simulink model "qiita2"  (R2019a)
settings: Solver=FixedStepDiscrete  StartTime=0.0  StopTime=Inf  FixedStep=0.001  RelTol=1e-3  EnableMultiTasking=on
libraries: mcp2515lib x13, simulink x13, robotlib x10, svdutilitieslib x1
settings Model: Creator=tatsuyai  LastModifiedBy=tatsuyai
settings SolverCC: PositivePriorityOrder=on
settings OptimizationCC: EnhancedBackFolding=on  PassReuseOutputArgsAs=Individual arguments  MaxStackSize=64  OptimizeBlockOrder=speed  DifferentSizesBufferReuse=on  OptimizationCustomize=off
settings DebuggingCC: ParameterTunabilityLossMsg=error
settings HardwareCC: ProdBitPerPointer=32  ProdBitPerSizeT=32  ProdBitPerPtrDiffT=32  ProdLargestAtomicInteger=Long  ProdLargestAtomicFloat=Double  ProdWordSize=32  ProdHWDeviceType=ARM Compatible->ARM Cortex  UseEmbeddedCoderFeatures=off  UseSimulinkCoderFeatures=off
settings SFSimCC: MATLABDynamicMemAlloc=off
settings RTWCC: SystemTargetFile=ert.tlc  HardwareBoard=Raspberry Pi - Robot Operating System (ROS)  TLCOptions="-aInlineSetEventsForThisBaseRateFcn=TLC_FALSE -aSuppressMultiTaskScheduler=TLC_FALSE  -aRateBasedStepFcn=0"  TemplateMakefile=ert_default_tmf  GenerateReport=on  Toolchain=Catkin  IncludeHyperlinkInReport=on  LaunchReport=on  TargetLang=C++  GenerateTraceInfo=on  GenerateTraceReport=on  GenerateTraceReportSl=on  GenerateTraceReportSf=on  GenerateTraceReportEml=on
settings CodeAppCC: ForceParamTrailComments=on  IgnoreCustomStorageClasses=off  OperatorAnnotations=on  SimulinkDataObjDesc=on  SFDataObjDesc=on  InsertBlockDesc=on
settings ERTTargetCC: SupportNonInlinedSFcns=on

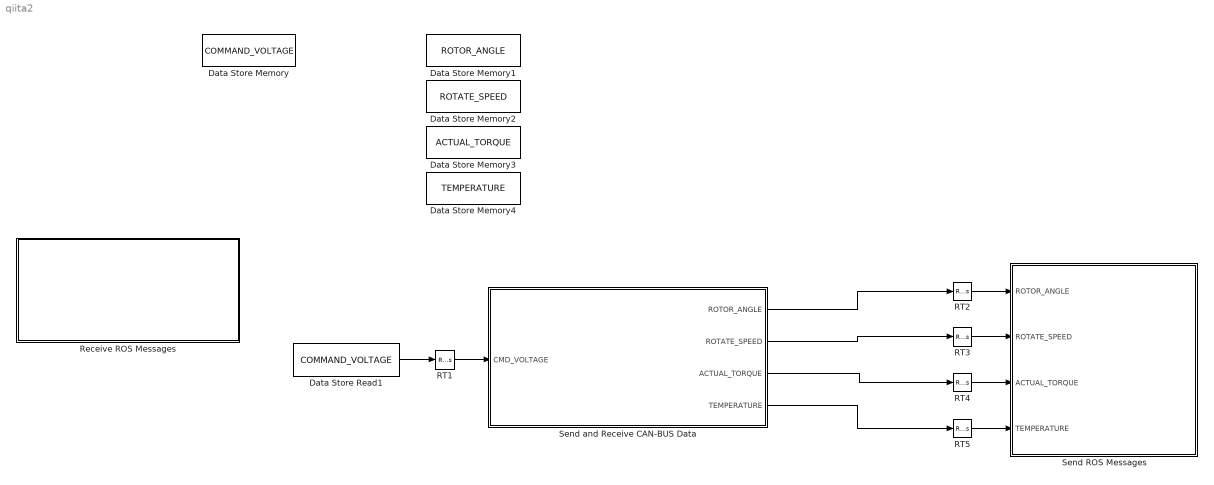
== system qiita2 ==
  Data Store Memory : DataStoreMemory  DataStoreName=COMMAND_VOLTAGE  ReadBeforeWriteMsg=warning  WriteAfterWriteMsg=warning  WriteAfterReadMsg=warning  ShowAdditionalParam=off
  Data Store Memory1 : DataStoreMemory  DataStoreName=ROTOR_ANGLE  ReadBeforeWriteMsg=warning  WriteAfterWriteMsg=warning  WriteAfterReadMsg=warning  ShowAdditionalParam=off
      settings: RTWStateStorageClass=ExportedGlobal
  Data Store Memory2 : DataStoreMemory  DataStoreName=ROTATE_SPEED  ReadBeforeWriteMsg=warning  WriteAfterWriteMsg=warning  WriteAfterReadMsg=warning  ShowAdditionalParam=off
      settings: RTWStateStorageClass=ExportedGlobal
  Data Store Memory3 : DataStoreMemory  DataStoreName=ACTUAL_TORQUE  ReadBeforeWriteMsg=warning  WriteAfterWriteMsg=warning  WriteAfterReadMsg=warning  ShowAdditionalParam=off
      settings: RTWStateStorageClass=ExportedGlobal
  Data Store Memory4 : DataStoreMemory  DataStoreName=TEMPERATURE  ReadBeforeWriteMsg=warning  WriteAfterWriteMsg=warning  WriteAfterReadMsg=warning  ShowAdditionalParam=off
      settings: RTWStateStorageClass=ExportedGlobal
  Data Store Read1 : DataStoreRead  DataStoreName=COMMAND_VOLTAGE
  RT1 : RateTransition  Deterministic=off  OutPortSampleTime=0.005
  RT{2..5} (4 alike) : RateTransition  Deterministic=off  OutPortSampleTime=0.01
  Receive ROS Messages : Subsystem  TreatAsAtomicUnit=on  SystemSampleTime=0.001
  Send ROS Messages : Subsystem  TreatAsAtomicUnit=on  SystemSampleTime=0.01
  Send and Receive CAN-BUS Data : Subsystem  TreatAsAtomicUnit=on  SystemSampleTime=0.005
  wires:
  RT3/1 -> Send ROS Messages/2(ROTATE_SPEED)
  RT1/1 -> Send and Receive CAN-BUS Data/1(CMD_VOLTAGE)
  Send and Receive CAN-BUS Data/1(ROTOR_ANGLE) -> RT2/1
  Data Store Read1/1 -> RT1/1
  RT2/1 -> Send ROS Messages/1(ROTOR_ANGLE)
  Send and Receive CAN-BUS Data/3(ACTUAL_TORQUE) -> RT4/1
  RT4/1 -> Send ROS Messages/3(ACTUAL_TORQUE)
  Send and Receive CAN-BUS Data/4(TEMPERATURE) -> RT5/1
  RT5/1 -> Send ROS Messages/4(TEMPERATURE)
  Send and Receive CAN-BUS Data/2(ROTATE_SPEED) -> RT3/1

== system qiita2/Receive ROS Messages ==
  Constant10 : Constant
  If Action Subsystem1 : Subsystem  TreatAsAtomicUnit=on
  If1 : If  IfExpression=u1 == 1  ShowElse=off
  Stop Simulation : Stop
  Subscribe : robotlib/Subscribe  topicSource=Specify your own  topic=/gm6020_1/cmd_voltage  messageType=std_msgs/Int16  sampleTime=-1  messageQueueLength=1
      settings: SourceProductName=ROS Toolbox
  Subsystem5 : Subsystem
  wires:
  Subscribe/2 -> If Action Subsystem1/1(In1)
  Subscribe/1 -> Subsystem5/2(RECEIVED), If1/1
  If1/1 -> If Action Subsystem1/Action
  Constant10/1 -> Subsystem5/1(TIMEOUT_LIMIT)

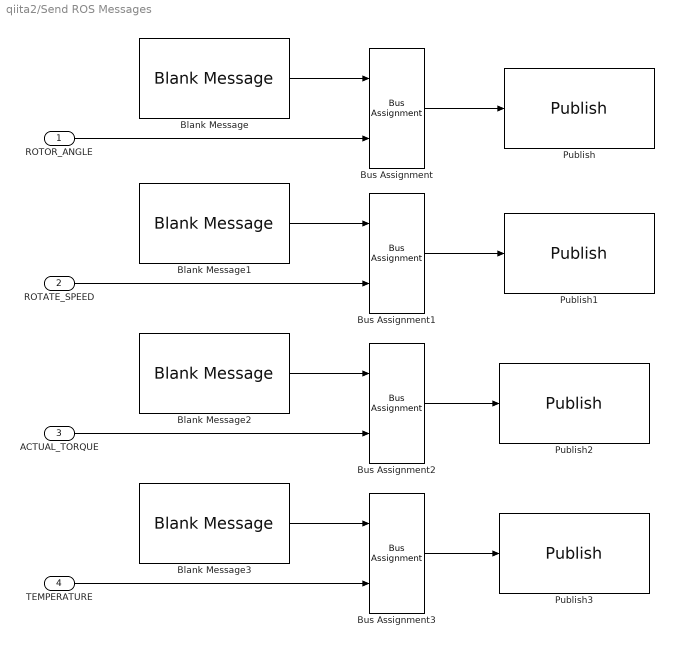
== system qiita2/Send ROS Messages ==
  ROTOR_ANGLE : Inport
  ROTATE_SPEED : Inport  Port=2
  ACTUAL_TORQUE : Inport  Port=3
  TEMPERATURE : Inport  Port=4
  Blank Message : robotlib/Blank Message  messageClass=Message  entityType=std_msgs/Float64  messageType=std_msgs/Float64  SampleTime=inf
      settings: SourceProductName=ROS Toolbox
  Blank Message1 : robotlib/Blank Message  messageClass=Message  entityType=std_msgs/Float64  messageType=std_msgs/Float64  SampleTime=inf
      settings: SourceProductName=ROS Toolbox
  Blank Message2 : robotlib/Blank Message  messageClass=Message  entityType=std_msgs/Float64  messageType=std_msgs/Float64  SampleTime=inf
      settings: SourceProductName=ROS Toolbox
  Blank Message3 : robotlib/Blank Message  messageClass=Message  entityType=std_msgs/Int8  messageType=std_msgs/Int8  SampleTime=inf
      settings: SourceProductName=ROS Toolbox
  Bus Assignment{,1..3} (4 alike) : BusAssignment  AssignedSignals=Data
  Publish : robotlib/Publish  topicSource=Specify your own  topic=/gm6020_1/rotor_angle  messageType=std_msgs/Float64  messageQueueLength=1
      settings: SourceProductName=ROS Toolbox
  Publish1 : robotlib/Publish  topicSource=Specify your own  topic=/gm6020_1/rotate_speed  messageType=std_msgs/Float64  messageQueueLength=1
      settings: SourceProductName=ROS Toolbox
  Publish2 : robotlib/Publish  topicSource=Specify your own  topic=/gm6020_1/actual_trq  messageType=std_msgs/Float64  messageQueueLength=1
      settings: SourceProductName=ROS Toolbox
  Publish3 : robotlib/Publish  topicSource=Specify your own  topic=/gm6020_1/temp  messageType=std_msgs/Int8  messageQueueLength=1
      settings: SourceProductName=ROS Toolbox
  wires:
  ROTOR_ANGLE/1 -> Bus Assignment/2
  Bus Assignment3/1 -> Publish3/1
  ACTUAL_TORQUE/1 -> Bus Assignment2/2
  Blank Message2/1 -> Bus Assignment2/1
  Bus Assignment/1 -> Publish/1
  ROTATE_SPEED/1 -> Bus Assignment1/2
  Blank Message/1 -> Bus Assignment/1
  Blank Message3/1 -> Bus Assignment3/1
  Bus Assignment2/1 -> Publish2/1
  Bus Assignment1/1 -> Publish1/1
  TEMPERATURE/1 -> Bus Assignment3/2
  Blank Message1/1 -> Bus Assignment1/1

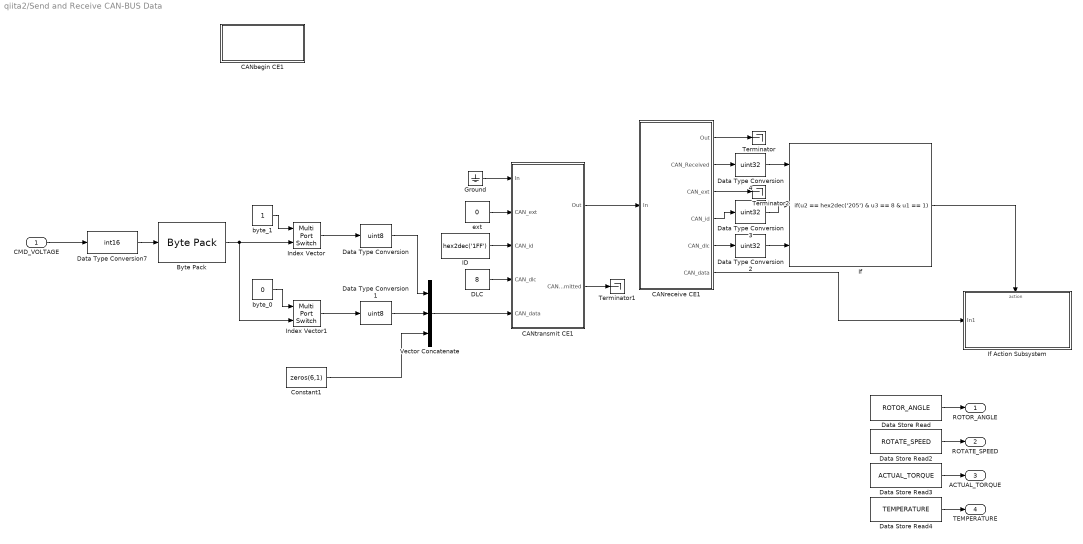
== system qiita2/Send and Receive CAN-BUS Data ==
  CMD_VOLTAGE : Inport
  Byte Pack : svdutilitieslib/Byte Pack  maskPackedDataType=uint8  datatypes={'int16'}  byteAlign=1  blockPlatform=arduinoert
      settings: SourceProductName=Embedded Coder Support Package for ARM Cortex-A Processors  SourceProductBaseCode=ECCORTEXA
  CANbegin CE1 : Subsystem  TreatAsAtomicUnit=on  mask{TargetHardware=Raspberry Pi, Oscillator=16, CANSpeed=1000, CSpin=10}
      mask prompts: TargetHardware "Target Hardware"; Oscillator "Oscillator frequency(MHz)"; CANSpeed "CAN speed(kHz)"; CSpin "Chip Select Pin"
      mask init:
      | % Get this mask's handle
      | maskObj = Simulink.Mask.get(gcb);
      | 
      | % Get the selected value from mask parameter's option
      | str_TargetHard = char(maskObj.Parameters(1).TypeOptions(TargetHardware));
      | str_Osc = char(maskObj.Parameters(2).TypeOptions(Oscillator));
      | str_CANSpeed = char(maskObj.Parameters(3).TypeOptions(CANSpeed));
      | 
      | % Set Icon
      | str1 = sprintf('%s(Model)',str_TargetHard);
      | str2 = sprintf('Oscillator: %s(MHz)',str_Osc);
      | str3 = sprintf('CAN Bus Speed: %s(kHz)',str_CANSpeed);
      | str4 = sprintf('Chip Select pin: %d',CSpin);
      | 
      | % Set the values of Variant Subsystem
      | switch str_TargetHard
      |     case 'Arduino'
      |         str = [str1,'\n',str2,'\n',str3,'\n',str4];
      |         evalin('base',sprintf('CSpin = %d;',CSpin));        
      |         evalin('base','Hardware = 1;');
      |     case 'Raspberry Pi'
      |         str = [str1,'\n',str2,'\n',str3];
      |         evalin('base',sprintf('clear CSpin',CSpin));           
      |         evalin('base','Hardware = 2;');     
      | end  
      | 
      | % Get the CAN Configuration register's value from mask parameter's option
      | if str_Osc == '8' %[MHz]
      |     switch str_CANSpeed
      |         case '1000'
      |             BPR = 0; PHSEG1 = 0; PRSEG = 0; PHSEG2 = 0;
      |         case '500'
      |             BPR = 0; PHSEG1 = 2; PRSEG = 0; PHSEG2 = 2;
      |         case '250'
      |             BPR = 0; PHSEG1 = 6; PRSEG = 0; PHSEG2 = 6;
      |         case '125'
      |             BPR = 1; PHSEG1 = 6; PRSEG = 1; PHSEG2 = 5;
      |         case '100'
      |             BPR = 1; PHSEG1 = 7; PRSEG = 2; PHSEG2 = 7;
      |         case '83.3'
      |             BPR = 1; PHSEG1 = 7; PRSEG = 6; PHSEG2 = 7;
      |         case '62.5'
      |             BPR = 3; PHSEG1 = 6; PRSEG = 0; PHSEG2 = 6;
      |         case '50'
      |             BPR = 3; PHSEG1 = 7; PRSEG = 2; PHSEG2 = 7;
      |         case '33.3'
      |             BPR = 4; PHSEG1 = 7; PRSEG = 6; PHSEG2 = 7;
      |     end            
      | elseif str_Osc == '16' %[MHz]
      |     switch str_CANSpeed  
      |         case '1000'
      |             BPR = 0; PHSEG1 = 2; PRSEG = 0; PHSEG2 = 2;
      |         case '500'
      |             BPR = 0; PHSEG1 = 6; PRSEG = 0; PHSEG2 = 6;
      |         case '250'
      |             BPR = 1; PHSEG1 = 6; PRSEG = 1; PHSEG2 = 5;        
      |         case '125'
      |             BPR = 3; PHSEG1 = 6; PRSEG = 0; PHSEG2 = 6;
      |         case '100'
      |             BPR = 3; PHSEG1 = 7; PRSEG = 2; PHSEG2 = 7;
      |         case '83.3'
      |             BPR = 3; PHSEG1 = 7; PRSEG = 6; PHSEG2 = 7;
      |         case '62.5'
      |             BPR = 7; PHSEG1 = 6; PRSEG = 0; PHSEG2 = 6;
      |         case '50'
      |             BPR = 7; PHSEG1 = 7; PRSEG = 2; PHSEG2 = 7;
      |         case '33.3'
      |             BPR = 9; PHSEG1 = 7; PRSEG = 6; PHSEG2 = 7;        
      |     end   
      | end
      | % Set the CAN Configuration register's value
      | address2A = BPR;          % bit7-6 :SJW, bit5-0: BPR
      | address29 = 192 ...       % bit7: BTLMODE = 1, bit6:SAM = 1
      |             + 8*PHSEG1 ...% bit5-3: PHSEG1
      |             +PRSEG;       % bit2-0: PRSEG
      | address28 = 128 ...       % bit7: SOF = 1, bit6:WAKFIL = 0
      |             + PHSEG2;     % bit5-3: 0, bit2-0: PHSEG2
      settings: RTWSystemCode=Nonreusable function
      mask TypeOptions TargetHardware: Arduino | Raspberry Pi
      mask Callback TargetHardware:
      | if(strcmp(get_param(gcb,'TargetHardware'),'Arduino'))
      |     set_param(gcb,'MaskVisibilities',{'on','on','on','on'})
      | else
      |     set_param(gcb,'MaskVisibilities',{'on','on','on','off'})
      | end
      mask TypeOptions Oscillator: 8 | 16
      mask TypeOptions CANSpeed: 1000 | 500 | 250 | 125 | 100 | 83.3 | 62.5 | 50 | 33.3
      mask DialogControl DescGroupVar Prompt: Description
      mask DialogControl DescTextVar Prompt: This block must be executed only once when beginning CAN communication because MCP2515’s register needs to be configured. And the frequency of oscillator for MCP2515 is also needed because it effects to the setting parameters of MCP2515's register.
      mask Display: disp(str)
  CANreceive CE1 : Subsystem  TreatAsAtomicUnit=on
      mask DialogControl DescGroupVar Prompt: Description
      mask DialogControl DescTextVar Prompt: CANreceive outputs CAN data by converting MCP2515 RX buffer register’s values. In/Out ports are no use because they are used for controlling the execution order. CAN_Received outputs 1(CAN received) or -1( No message).
  CANtransmit CE1 : Subsystem  TreatAsAtomicUnit=on
      mask DialogControl DescGroupVar Prompt: Description
      mask DialogControl DescTextVar Prompt: CANtransmit inputs CAN data by converting MCP2515 TX buffer register’s values. In/Out ports are no use because they are used for controlling the execution order. CAN_Transmitted outputs 1(Success) or 2(Fail).
  Constant1 : Constant  Value=zeros(6,1)  OutDataTypeStr=uint8
  DLC : Constant  Value=8  OutDataTypeStr=uint8
  Data Store Read : DataStoreRead  DataStoreName=ROTOR_ANGLE
  Data Store Read2 : DataStoreRead  DataStoreName=ROTATE_SPEED
  Data Store Read3 : DataStoreRead  DataStoreName=ACTUAL_TORQUE
  Data Store Read4 : DataStoreRead  DataStoreName=TEMPERATURE
  Data Type Conversion : DataTypeConversion  OutDataTypeStr=uint8
  Data Type Conversion1 : DataTypeConversion  OutDataTypeStr=uint8
  Data Type Conversion2 : DataTypeConversion  OutDataTypeStr=uint32
  Data Type Conversion3 : DataTypeConversion  OutDataTypeStr=uint32
  Data Type Conversion4 : DataTypeConversion  OutDataTypeStr=uint32
  Data Type Conversion7 : DataTypeConversion  OutDataTypeStr=int16
  Ground : Ground
  ID : Constant  Value=hex2dec('1FF')  OutDataTypeStr=uint32
  If : If  NumInputs=3  IfExpression=u2 == hex2dec('205') & u3 == 8 & u1 == 1  ShowElse=off
  If Action Subsystem : Subsystem  TreatAsAtomicUnit=on
  Index Vector : MultiPortSwitch  DataPortOrder=Zero-based contiguous  Inputs=1  zeroidx=on
  Index Vector1 : MultiPortSwitch  DataPortOrder=Zero-based contiguous  Inputs=1  zeroidx=on
  Terminator : Terminator
  Terminator1 : Terminator
  Terminator2 : Terminator
  Vector Concatenate : Concatenate  NumInputs=3
  byte_0 : Constant  Value=0  OutDataTypeStr=uint8
  byte_1 : Constant  OutDataTypeStr=uint8
  ext : Constant  Value=0  OutDataTypeStr=uint8
  ROTOR_ANGLE : Outport
  ROTATE_SPEED : Outport  Port=2
  ACTUAL_TORQUE : Outport  Port=3
  TEMPERATURE : Outport  Port=4
  wires:
  CANreceive CE1/6(CAN_data) -> If Action Subsystem/1(In1)
  Data Type Conversion/1 -> Vector Concatenate/1
  If/1 -> If Action Subsystem/Action
  Constant1/1 -> Vector Concatenate/3
  CANtransmit CE1/2(CAN_Transmitted) -> Terminator1/1
  CANreceive CE1/3(CAN_ext) -> Terminator2/1
  CANreceive CE1/2(CAN_Received) -> Data Type Conversion4/1
  Data Type Conversion2/1 -> If/3
  CANreceive CE1/4(CAN_id) -> Data Type Conversion3/1
  Vector Concatenate/1 -> CANtransmit CE1/5(CAN_data)
  byte_1/1 -> Index Vector/1
  ID/1 -> CANtransmit CE1/3(CAN_id)
  CANreceive CE1/1(Out) -> Terminator/1
  byte_0/1 -> Index Vector1/1
  Data Type Conversion7/1 -> Byte Pack/1
  CANreceive CE1/5(CAN_dlc) -> Data Type Conversion2/1
  ext/1 -> CANtransmit CE1/2(CAN_ext)
  Data Type Conversion4/1 -> If/1
  Ground/1 -> CANtransmit CE1/1(In)
  Index Vector1/1 -> Data Type Conversion1/1
  Index Vector/1 -> Data Type Conversion/1
  Byte Pack/1 -> Index Vector1/2, Index Vector/2
  CANtransmit CE1/1(Out) -> CANreceive CE1/1(In)
  DLC/1 -> CANtransmit CE1/4(CAN_dlc)
  Data Type Conversion1/1 -> Vector Concatenate/2
  Data Type Conversion3/1 -> If/2
  CMD_VOLTAGE/1 -> Data Type Conversion7/1
  Data Store Read/1 -> ROTOR_ANGLE/1
  Data Store Read3/1 -> ACTUAL_TORQUE/1
  Data Store Read4/1 -> TEMPERATURE/1
  Data Store Read2/1 -> ROTATE_SPEED/1

== system qiita2/Receive ROS Messages/If Action Subsystem1 ==
  In1 : Inport
  Action Port : ActionPort  ActionPortLabel=if(u1 == 1)
  Bus Selector : BusSelector  OutputSignals=Data
  Data Store Write : DataStoreWrite  DataStoreName=COMMAND_VOLTAGE
  wires:
  In1/1 -> Bus Selector/1
  Bus Selector/1 -> Data Store Write/1  "<Data>"

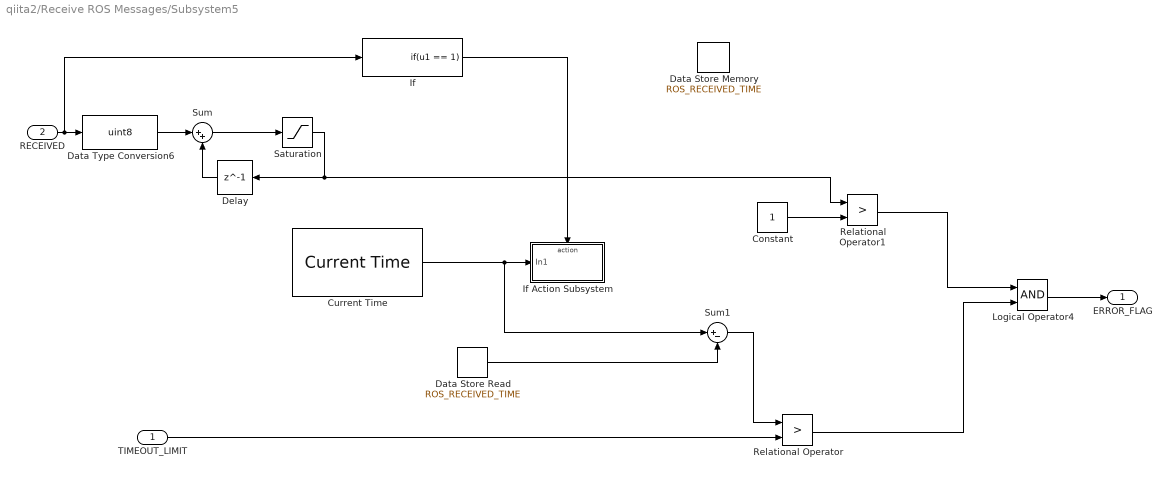
== system qiita2/Receive ROS Messages/Subsystem5 ==
  TIMEOUT_LIMIT : Inport
  RECEIVED : Inport  Port=2
  Constant : Constant
  Current Time : robotlib/Current Time  OutputFormat=double  SampleTime=-1  ModelName=qiita2
      settings: SourceProductName=Robotics System Toolbox  SourceProductBaseCode=RO
  Data Store Memory : DataStoreMemory  DataStoreName=ROS_RECEIVED_TIME  ReadBeforeWriteMsg=warning  WriteAfterWriteMsg=warning  WriteAfterReadMsg=warning  InitialValue=10  ShowAdditionalParam=off
  Data Store Read : DataStoreRead  DataStoreName=ROS_RECEIVED_TIME
  Data Type Conversion6 : DataTypeConversion  OutDataTypeStr=uint8
  Delay : Delay  DelayLength=1
  If : If  IfExpression=u1 == 1  ShowElse=off
  If Action Subsystem : Subsystem  TreatAsAtomicUnit=on
  Logical Operator4 : Logic  AllPortsSameDT=off  OutDataTypeStr=boolean
  Relational Operator : RelationalOperator  Operator=>  OutDataTypeStr=boolean  RndMeth=Simplest
  Relational Operator1 : RelationalOperator  Operator=>  OutDataTypeStr=boolean  RndMeth=Simplest
  Saturation : Saturate  UpperLimit=2  LowerLimit=0
  Sum : Sum  Inputs=|++
  Sum1 : Sum  Inputs=|+-
  ERROR_FLAG : Outport
  wires:
  Data Store Read/1 -> Sum1/2
  Sum1/1 -> Relational Operator/1
  RECEIVED/1 -> If/1, Data Type Conversion6/1
  Current Time/1 -> Sum1/1, If Action Subsystem/1(In1)
  If/1 -> If Action Subsystem/Action
  TIMEOUT_LIMIT/1 -> Relational Operator/2
  Relational Operator/1 -> Logical Operator4/2
  Saturation/1 -> Delay/1, Relational Operator1/1
  Sum/1 -> Saturation/1
  Delay/1 -> Sum/2
  Constant/1 -> Relational Operator1/2
  Logical Operator4/1 -> ERROR_FLAG/1
  Relational Operator1/1 -> Logical Operator4/1
  Data Type Conversion6/1 -> Sum/1

== system qiita2/Send and Receive CAN-BUS Data/CANbegin CE1 ==
  Constant : Constant  Value=0  OutDataTypeStr=boolean  SampleTime=-1
  Temporary buffer : DataStoreMemory  DataStoreName=temp_1byte  ReadBeforeWriteMsg=warning  WriteAfterWriteMsg=warning  WriteAfterReadMsg=warning  ShowAdditionalParam=off  OutDataTypeStr=uint8
  Unit Delay : UnitDelay  InitialCondition=1  SampleTime=-1  HasFrameUpgradeWarning=on
  setup : Subsystem  TreatAsAtomicUnit=on
      settings: RTWSystemCode=Nonreusable function  RTWFileNameOpts=Use subsystem name
  wires:
  Unit Delay/1 -> setup/Enable
  Constant/1 -> Unit Delay/1

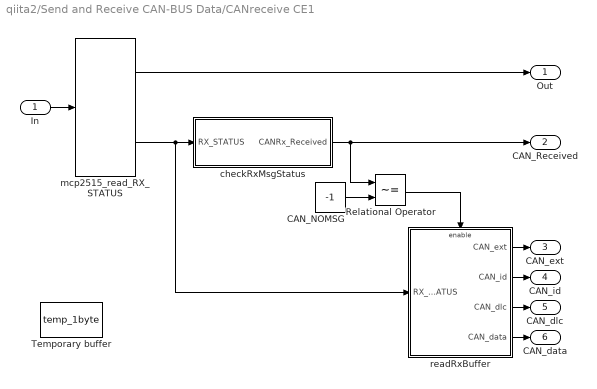
== system qiita2/Send and Receive CAN-BUS Data/CANreceive CE1 ==
  In : Inport
  CAN_NOMSG : Constant  Value=-1  OutDataTypeStr=int8
  Relational Operator : RelationalOperator  Operator=~=  OutDataTypeStr=boolean  RndMeth=Nearest
  Temporary buffer : DataStoreMemory  DataStoreName=temp_1byte  ReadBeforeWriteMsg=warning  WriteAfterWriteMsg=warning  WriteAfterReadMsg=warning  ShowAdditionalParam=off  OutDataTypeStr=uint8
  checkRxMsgStatus : Subsystem  TreatAsAtomicUnit=on
  mcp2515_read_RX_STATUS : mcp2515lib/CAN application/mcp2515 driver CE1/mcp2515_read_RX_STATUS  SystemSampleTime=-1
      settings: SourceProductName=CAN device driver for mcp2515
  readRxBuffer : Subsystem  TreatAsAtomicUnit=on
  Out : Outport
  CAN_Received : Outport  Port=2
  CAN_ext : Outport  Port=3
  CAN_id : Outport  Port=4
  CAN_dlc : Outport  Port=5
  CAN_data : Outport  Port=6
  wires:
  In/1 -> mcp2515_read_RX_STATUS/1
  mcp2515_read_RX_STATUS/1 -> Out/1
  checkRxMsgStatus/1(CANRx_Received) -> CAN_Received/1, Relational Operator/1
  mcp2515_read_RX_STATUS/2 -> readRxBuffer/1(RX_STATUS), checkRxMsgStatus/1(RX_STATUS)
  readRxBuffer/1(CAN_ext) -> CAN_ext/1
  readRxBuffer/2(CAN_id) -> CAN_id/1
  readRxBuffer/3(CAN_dlc) -> CAN_dlc/1
  readRxBuffer/4(CAN_data) -> CAN_data/1
  CAN_NOMSG/1 -> Relational Operator/2
  Relational Operator/1 -> readRxBuffer/Enable

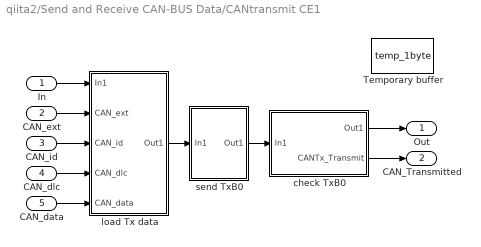
== system qiita2/Send and Receive CAN-BUS Data/CANtransmit CE1 ==
  In : Inport
  CAN_ext : Inport  Port=2
  CAN_id : Inport  Port=3
  CAN_dlc : Inport  Port=4
  CAN_data : Inport  Port=5
  Temporary buffer : DataStoreMemory  DataStoreName=temp_1byte  ReadBeforeWriteMsg=warning  WriteAfterWriteMsg=warning  WriteAfterReadMsg=warning  ShowAdditionalParam=off  OutDataTypeStr=uint8
  check TxB0 : Subsystem  TreatAsAtomicUnit=on
  load Tx data : Subsystem  TreatAsAtomicUnit=on
  send TxB0 : Subsystem  TreatAsAtomicUnit=on
  Out : Outport
  CAN_Transmitted : Outport  Port=2
  wires:
  In/1 -> load Tx data/1(In1)
  load Tx data/1(Out1) -> send TxB0/1(In1)
  send TxB0/1(Out1) -> check TxB0/1(In1)
  check TxB0/1(Out1) -> Out/1
  check TxB0/2(CANTx_Transmit) -> CAN_Transmitted/1
  CAN_ext/1 -> load Tx data/2(CAN_ext)
  CAN_id/1 -> load Tx data/3(CAN_id)
  CAN_dlc/1 -> load Tx data/4(CAN_dlc)
  CAN_data/1 -> load Tx data/5(CAN_data)

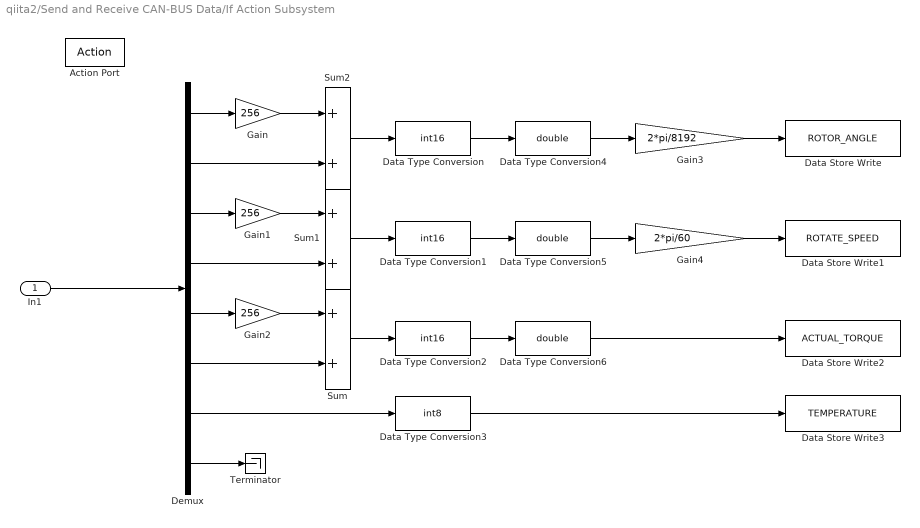
== system qiita2/Send and Receive CAN-BUS Data/If Action Subsystem ==
  In1 : Inport
  Action Port : ActionPort  ActionPortLabel=if(u2 == hex2dec('205') & u3 == 8 & u1 == 1)
  Data Store Write : DataStoreWrite  DataStoreName=ROTOR_ANGLE
  Data Store Write1 : DataStoreWrite  DataStoreName=ROTATE_SPEED
  Data Store Write2 : DataStoreWrite  DataStoreName=ACTUAL_TORQUE
  Data Store Write3 : DataStoreWrite  DataStoreName=TEMPERATURE
  Data Type Conversion : DataTypeConversion  OutDataTypeStr=int16
  Data Type Conversion1 : DataTypeConversion  OutDataTypeStr=int16
  Data Type Conversion2 : DataTypeConversion  OutDataTypeStr=int16
  Data Type Conversion3 : DataTypeConversion  OutDataTypeStr=int8
  Data Type Conversion4 : DataTypeConversion  OutDataTypeStr=double
  Data Type Conversion5 : DataTypeConversion  OutDataTypeStr=double
  Data Type Conversion6 : DataTypeConversion  OutDataTypeStr=double
  Demux : Demux  Outputs=8
  Gain : Gain  Gain=256
  Gain1 : Gain  Gain=256
  Gain2 : Gain  Gain=256
  Gain3 : Gain  Gain=2*pi/8192
  Gain4 : Gain  Gain=2*pi/60
  Sum : Sum
  Sum1 : Sum
  Sum2 : Sum
  Terminator : Terminator
  wires:
  In1/1 -> Demux/1
  Demux/1 -> Gain/1
  Demux/3 -> Gain1/1
  Demux/5 -> Gain2/1
  Demux/8 -> Terminator/1
  Gain2/1 -> Sum/1
  Demux/6 -> Sum/2
  Gain/1 -> Sum2/1
  Gain1/1 -> Sum1/1
  Demux/2 -> Sum2/2
  Demux/4 -> Sum1/2
  Sum2/1 -> Data Type Conversion/1
  Sum/1 -> Data Type Conversion2/1
  Sum1/1 -> Data Type Conversion1/1
  Data Type Conversion/1 -> Data Type Conversion4/1
  Data Type Conversion1/1 -> Data Type Conversion5/1
  Data Type Conversion2/1 -> Data Type Conversion6/1
  Demux/7 -> Data Type Conversion3/1
  Data Type Conversion3/1 -> Data Store Write3/1
  Data Type Conversion6/1 -> Data Store Write2/1
  Data Type Conversion5/1 -> Gain4/1
  Data Type Conversion4/1 -> Gain3/1
  Gain3/1 -> Data Store Write/1
  Gain4/1 -> Data Store Write1/1

== system qiita2/Receive ROS Messages/Subsystem5/If Action Subsystem ==
  In1 : Inport
  Action Port : ActionPort  ActionPortLabel=if(u1 == 1)
  Data Store Write : DataStoreWrite  DataStoreName=ROS_RECEIVED_TIME
  wires:
  In1/1 -> Data Store Write/1

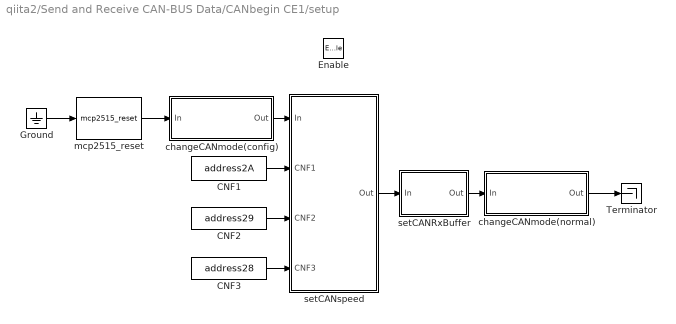
== system qiita2/Send and Receive CAN-BUS Data/CANbegin CE1/setup ==
  Enable : EnablePort
  CNF1 : Constant  Value=address2A  OutDataTypeStr=uint8
  CNF2 : Constant  Value=address29  OutDataTypeStr=uint8
  CNF3 : Constant  Value=address28  OutDataTypeStr=uint8
  Ground : Ground
  Terminator : Terminator
  changeCANmode(config) : Subsystem  TreatAsAtomicUnit=on
  changeCANmode(normal) : Subsystem  TreatAsAtomicUnit=on
  mcp2515_reset : mcp2515lib/CAN application/mcp2515 driver CE1/mcp2515_reset  SystemSampleTime=-1
      settings: SourceProductName=CAN device driver for mcp2515
  setCANRxBuffer : Subsystem  TreatAsAtomicUnit=on
  setCANspeed : Subsystem  TreatAsAtomicUnit=on
  wires:
  CNF3/1 -> setCANspeed/4(CNF3)
  CNF2/1 -> setCANspeed/3(CNF2)
  CNF1/1 -> setCANspeed/2(CNF1)
  mcp2515_reset/1 -> changeCANmode(config)/1(In)
  changeCANmode(config)/1(Out) -> setCANspeed/1(In)
  setCANspeed/1(Out) -> setCANRxBuffer/1(In)
  setCANRxBuffer/1(Out) -> changeCANmode(normal)/1(In)
  Ground/1 -> mcp2515_reset/1
  changeCANmode(normal)/1(Out) -> Terminator/1

== system qiita2/Send and Receive CAN-BUS Data/CANreceive CE1/checkRxMsgStatus ==
  RX_STATUS : Inport
  Bitmask_RxBn : simulink/Logic and Bit Operations/Bitwise Operator  logicop=AND  UseBitMask=on  BitMask=bin2dec('11000000')  BitMaskRealWorld=Stored Integer
  CAN_NOMSG : Constant  Value=-1  OutDataTypeStr=int8
  CAN_OK : Constant  OutDataTypeStr=int8
  Switch : Switch  Criteria=u2 > Threshold
  CANRx_Received : Outport
  wires:
  RX_STATUS/1 -> Bitmask_RxBn/1
  CAN_OK/1 -> Switch/1
  CAN_NOMSG/1 -> Switch/3
  Switch/1 -> CANRx_Received/1
  Bitmask_RxBn/1 -> Switch/2

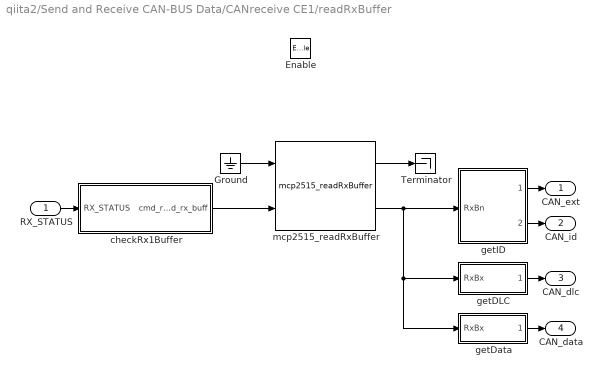
== system qiita2/Send and Receive CAN-BUS Data/CANreceive CE1/readRxBuffer ==
  RX_STATUS : Inport
  Enable : EnablePort
  Ground : Ground
  Terminator : Terminator
  checkRx1Buffer : Subsystem  TreatAsAtomicUnit=on
  getDLC : Subsystem  TreatAsAtomicUnit=on
  getData : Subsystem  TreatAsAtomicUnit=on
  getID : Subsystem  TreatAsAtomicUnit=on
      settings: RTWSystemCode=Inline
  mcp2515_readRxBuffer : mcp2515lib/CAN application/mcp2515 driver CE1/mcp2515_readRxBuffer  SystemSampleTime=-1
      settings: SourceProductName=CAN device driver for mcp2515
  CAN_ext : Outport
  CAN_id : Outport  Port=2
  CAN_dlc : Outport  Port=3
  CAN_data : Outport  Port=4
  wires:
  getData/1(CAN_data) -> CAN_data/1
  mcp2515_readRxBuffer/2 -> getID/1(RxBn), getData/1(RxBx), getDLC/1(RxBx)
  getID/2(CAN_id) -> CAN_id/1
  getID/1(CAN_ext) -> CAN_ext/1
  getDLC/1(CAN_dlc) -> CAN_dlc/1
  mcp2515_readRxBuffer/1 -> Terminator/1
  Ground/1 -> mcp2515_readRxBuffer/1
  RX_STATUS/1 -> checkRx1Buffer/1(RX_STATUS)
  checkRx1Buffer/1(cmd_read_rx_buff) -> mcp2515_readRxBuffer/2

== system qiita2/Send and Receive CAN-BUS Data/CANtransmit CE1/check TxB0 ==
  In1 : Inport
  Bitmask_TxReq : simulink/Logic and Bit Operations/Bitwise Operator  logicop=AND  UseBitMask=on  BitMask=bin2dec('00001000')  BitMaskRealWorld=Stored Integer
  CAN_FAIL : Constant  Value=2  OutDataTypeStr=int8
  CAN_OK : Constant  OutDataTypeStr=int8
  MCP_TxB0CTRL1 : Constant  Value=hex2dec('30')  OutDataTypeStr=uint8
  Switch : Switch  Criteria=u2 > Threshold
  mcp2515_readRegister : mcp2515lib/CAN application/mcp2515 driver CE1/mcp2515_readRegister  SystemSampleTime=-1
      settings: SourceProductName=CAN device driver for mcp2515
  Out1 : Outport
  CANTx_Transmit : Outport  Port=2
  wires:
  CAN_FAIL/1 -> Switch/3
  mcp2515_readRegister/1 -> Out1/1
  mcp2515_readRegister/2 -> Bitmask_TxReq/1
  MCP_TxB0CTRL1/1 -> mcp2515_readRegister/2
  Bitmask_TxReq/1 -> Switch/2
  Switch/1 -> CANTx_Transmit/1
  CAN_OK/1 -> Switch/1
  In1/1 -> mcp2515_readRegister/1

== system qiita2/Send and Receive CAN-BUS Data/CANtransmit CE1/load Tx data ==
  In1 : Inport
  CAN_ext : Inport  Port=2
  CAN_id : Inport  Port=3
  CAN_dlc : Inport  Port=4
  CAN_data : Inport  Port=5
  MCP_load_TxB0 : Constant  Value=hex2dec('40')  OutDataTypeStr=uint8
  Vector Concatenate : Concatenate  NumInputs=3
  mcp2515_writeTxBuffer : mcp2515lib/CAN application/mcp2515 driver CE1/mcp2515_writeTxBuffer  SystemSampleTime=-1
      settings: SourceProductName=CAN device driver for mcp2515
  setID : Subsystem  TreatAsAtomicUnit=on
      settings: RTWSystemCode=Inline
  Out1 : Outport
  wires:
  CAN_ext/1 -> setID/1(ext)
  CAN_id/1 -> setID/2(id)
  CAN_data/1 -> Vector Concatenate/3
  CAN_dlc/1 -> Vector Concatenate/2
  setID/1(TxBn_ID) -> Vector Concatenate/1
  In1/1 -> mcp2515_writeTxBuffer/1
  mcp2515_writeTxBuffer/1 -> Out1/1
  MCP_load_TxB0/1 -> mcp2515_writeTxBuffer/2
  Vector Concatenate/1 -> mcp2515_writeTxBuffer/3

== system qiita2/Send and Receive CAN-BUS Data/CANtransmit CE1/send TxB0 ==
  In1 : Inport
  MCP_TxB0CTRL : Constant  Value=hex2dec('30')  OutDataTypeStr=uint8
  TxREQ : Constant  Value=8  OutDataTypeStr=uint8
  mcp2515_writeRegister1 : mcp2515lib/CAN application/mcp2515 driver CE1/mcp2515_writeRegister  SystemSampleTime=-1
      settings: SourceProductName=CAN device driver for mcp2515
  Out1 : Outport
  wires:
  MCP_TxB0CTRL/1 -> mcp2515_writeRegister1/2
  mcp2515_writeRegister1/1 -> Out1/1
  In1/1 -> mcp2515_writeRegister1/1
  TxREQ/1 -> mcp2515_writeRegister1/3

== system qiita2/Send and Receive CAN-BUS Data/CANbegin CE1/setup/changeCANmode(config) ==
  In : Inport
  MCP_CANCTRL : Constant  Value=hex2dec('0F')  OutDataTypeStr=uint8
  MODE_CONFIG : Constant  Value=hex2dec('80')  OutDataTypeStr=uint8
  MODE_MASK : Constant  Value=hex2dec('E0')  OutDataTypeStr=uint8
  mcp2515_modifyRegister : mcp2515lib/CAN application/mcp2515 driver CE1/mcp2515_modifyRegister  SystemSampleTime=-1
      settings: SourceProductName=CAN device driver for mcp2515
  Out : Outport
  wires:
  MODE_CONFIG/1 -> mcp2515_modifyRegister/4
  MODE_MASK/1 -> mcp2515_modifyRegister/3
  MCP_CANCTRL/1 -> mcp2515_modifyRegister/2
  In/1 -> mcp2515_modifyRegister/1
  mcp2515_modifyRegister/1 -> Out/1

== system qiita2/Send and Receive CAN-BUS Data/CANbegin CE1/setup/changeCANmode(normal) ==
  In : Inport
  MCP_CANCTRL : Constant  Value=hex2dec('0F')  OutDataTypeStr=uint8
  MODE_MASK : Constant  Value=hex2dec('E0')  OutDataTypeStr=uint8
  MODE_NORMAL : Constant  Value=0  OutDataTypeStr=uint8
  mcp2515_modifyRegister : mcp2515lib/CAN application/mcp2515 driver CE1/mcp2515_modifyRegister  SystemSampleTime=-1
      settings: SourceProductName=CAN device driver for mcp2515
  Out : Outport
  wires:
  MODE_MASK/1 -> mcp2515_modifyRegister/3
  MODE_NORMAL/1 -> mcp2515_modifyRegister/4
  MCP_CANCTRL/1 -> mcp2515_modifyRegister/2
  In/1 -> mcp2515_modifyRegister/1
  mcp2515_modifyRegister/1 -> Out/1

== system qiita2/Send and Receive CAN-BUS Data/CANbegin CE1/setup/setCANRxBuffer ==
  note: RXB0
  note: RXB1
  note: no filter, no mask
  In : Inport
  MCP_RXB0CTRL : Constant  Value=hex2dec('60')  OutDataTypeStr=uint8
  MCP_RXB1CTRL : Constant  Value=hex2dec('70')  OutDataTypeStr=uint8
  MCP_RXB_RX_MASK : Constant  Value=hex2dec('60')  OutDataTypeStr=uint8
  mcp2515_writeRegister : mcp2515lib/CAN application/mcp2515 driver CE1/mcp2515_writeRegister  SystemSampleTime=-1
      settings: SourceProductName=CAN device driver for mcp2515
  mcp2515_writeRegister1 : mcp2515lib/CAN application/mcp2515 driver CE1/mcp2515_writeRegister  SystemSampleTime=-1
      settings: SourceProductName=CAN device driver for mcp2515
  Out : Outport
  wires:
  MCP_RXB0CTRL/1 -> mcp2515_writeRegister/2
  MCP_RXB1CTRL/1 -> mcp2515_writeRegister1/2
  MCP_RXB_RX_MASK/1 -> mcp2515_writeRegister/3, mcp2515_writeRegister1/3
  In/1 -> mcp2515_writeRegister/1
  mcp2515_writeRegister1/1 -> Out/1
  mcp2515_writeRegister/1 -> mcp2515_writeRegister1/1

== system qiita2/Send and Receive CAN-BUS Data/CANbegin CE1/setup/setCANspeed ==
  In : Inport
  CNF1 : Inport  Port=2
  CNF2 : Inport  Port=3
  CNF3 : Inport  Port=4
  MCP_CNF1 : Constant  Value=hex2dec('2A')  OutDataTypeStr=uint8
  MCP_CNF2 : Constant  Value=hex2dec('29')  OutDataTypeStr=uint8
  MCP_CNF3 : Constant  Value=hex2dec('28')  OutDataTypeStr=uint8
  mcp2515_writeRegister : mcp2515lib/CAN application/mcp2515 driver CE1/mcp2515_writeRegister  SystemSampleTime=-1
      settings: SourceProductName=CAN device driver for mcp2515
  mcp2515_writeRegister1 : mcp2515lib/CAN application/mcp2515 driver CE1/mcp2515_writeRegister  SystemSampleTime=-1
      settings: SourceProductName=CAN device driver for mcp2515
  mcp2515_writeRegister2 : mcp2515lib/CAN application/mcp2515 driver CE1/mcp2515_writeRegister  SystemSampleTime=-1
      settings: SourceProductName=CAN device driver for mcp2515
  Out : Outport
  wires:
  MCP_CNF2/1 -> mcp2515_writeRegister1/2
  MCP_CNF3/1 -> mcp2515_writeRegister2/2
  CNF3/1 -> mcp2515_writeRegister2/3
  CNF1/1 -> mcp2515_writeRegister/3
  MCP_CNF1/1 -> mcp2515_writeRegister/2
  CNF2/1 -> mcp2515_writeRegister1/3
  In/1 -> mcp2515_writeRegister/1
  mcp2515_writeRegister/1 -> mcp2515_writeRegister1/1
  mcp2515_writeRegister1/1 -> mcp2515_writeRegister2/1
  mcp2515_writeRegister2/1 -> Out/1

== system qiita2/Send and Receive CAN-BUS Data/CANreceive CE1/readRxBuffer/checkRx1Buffer ==
  RX_STATUS : Inport
  Bitmask_RxB1_Status : simulink/Logic and Bit Operations/Bitwise Operator  logicop=AND  UseBitMask=on  BitMask=bin2dec('10000000')  BitMaskRealWorld=Stored Integer
  MCP_READ_RxB0 : Constant  Value=hex2dec('90')  OutDataTypeStr=uint8
  MCP_READ_RxB1 : Constant  Value=hex2dec('94')  OutDataTypeStr=uint8
  Switch : Switch  Criteria=u2 > Threshold
  cmd_read_rx_buff : Outport
  wires:
  Switch/1 -> cmd_read_rx_buff/1
  MCP_READ_RxB1/1 -> Switch/1
  MCP_READ_RxB0/1 -> Switch/3
  Bitmask_RxB1_Status/1 -> Switch/2
  RX_STATUS/1 -> Bitmask_RxB1_Status/1

== system qiita2/Send and Receive CAN-BUS Data/CANreceive CE1/readRxBuffer/getDLC ==
  RxBx : Inport
  Bitwise Operator : simulink/Logic and Bit Operations/Bitwise Operator  logicop=AND  UseBitMask=off  NumInputPorts=2  BitMask=bin2dec('11011001')  BitMaskRealWorld=Stored Integer
  MCP_DLC_MASK : Constant  Value=hex2dec('0F')  OutDataTypeStr=uint8
  RxDLC : Selector  IndexMode=Zero-based  InputPortWidth=13  IndexOptions=Index vector (dialog)  Indices=4  OutputSizes=1
  CAN_dlc : Outport
  wires:
  Bitwise Operator/1 -> CAN_dlc/1
  RxBx/1 -> RxDLC/1
  RxDLC/1 -> Bitwise Operator/1
  MCP_DLC_MASK/1 -> Bitwise Operator/2

== system qiita2/Send and Receive CAN-BUS Data/CANreceive CE1/readRxBuffer/getData ==
  RxBx : Inport
  RxData : Selector  IndexMode=Zero-based  InputPortWidth=13  IndexOptions=Index vector (dialog)  Indices=[5:12]  OutputSizes=1
  CAN_data : Outport
  wires:
  RxBx/1 -> RxData/1
  RxData/1 -> CAN_data/1

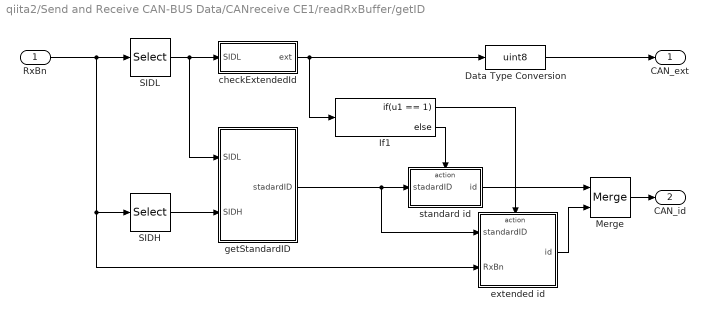
== system qiita2/Send and Receive CAN-BUS Data/CANreceive CE1/readRxBuffer/getID ==
  RxBn : Inport
  Data Type Conversion : DataTypeConversion  OutDataTypeStr=uint8  RndMeth=Simplest
  If1 : If  IfExpression=u1 == 1
  Merge : Merge
  SIDH : Selector  IndexMode=Zero-based  InputPortWidth=13  IndexOptions=Index vector (dialog)  Indices=0  OutputSizes=1
  SIDL : Selector  IndexMode=Zero-based  InputPortWidth=13  IndexOptions=Index vector (dialog)  Indices=1  OutputSizes=1
  checkExtendedId : Subsystem
  extended id : Subsystem  TreatAsAtomicUnit=on
      settings: RTWSystemCode=Inline
  getStandardID : Subsystem
  standard id : Subsystem  TreatAsAtomicUnit=on
      settings: RTWSystemCode=Inline
  CAN_ext : Outport
  CAN_id : Outport  Port=2
  wires:
  standard id/1(id) -> Merge/1
  extended id/1(id) -> Merge/2
  Merge/1 -> CAN_id/1
  If1/2 -> standard id/Action
  If1/1 -> extended id/Action
  RxBn/1 -> extended id/2(RxBn), SIDH/1, SIDL/1
  getStandardID/1(stadardID) -> standard id/1(stadardID), extended id/1(standardID)
  SIDL/1 -> getStandardID/1(SIDL), checkExtendedId/1(SIDL)
  SIDH/1 -> getStandardID/2(SIDH)
  checkExtendedId/1(ext) -> Data Type Conversion/1, If1/1
  Data Type Conversion/1 -> CAN_ext/1

== system qiita2/Send and Receive CAN-BUS Data/CANtransmit CE1/load Tx data/setID ==
  ext : Inport
  id : Inport  Port=2
  Extended ID : Subsystem  TreatAsAtomicUnit=on
  If : If
  Merge : Merge
  Standard ID : Subsystem  TreatAsAtomicUnit=on
  TxBn_ID : Outport
  wires:
  ext/1 -> If/1
  If/1 -> Extended ID/Action
  If/2 -> Standard ID/Action
  Extended ID/1(TxBn_ID) -> Merge/2
  Standard ID/1(TxBn_ID) -> Merge/1
  Merge/1 -> TxBn_ID/1
  id/1 -> Extended ID/1(id), Standard ID/1(id)

== system qiita2/Send and Receive CAN-BUS Data/CANreceive CE1/readRxBuffer/getID/checkExtendedId ==
  SIDL : Inport
  Bitmask_EXIDE : simulink/Logic and Bit Operations/Bitwise Operator  logicop=AND  UseBitMask=on  BitMask=bin2dec('00001000')  BitMaskRealWorld=Stored Integer
  MCP_TXB_EXIDE_M : Constant  Value=hex2dec('08')  OutDataTypeStr=uint8
  Relational Operator : RelationalOperator  Operator===  OutDataTypeStr=boolean  RndMeth=Nearest
  ext : Outport
  wires:
  Relational Operator/1 -> ext/1
  MCP_TXB_EXIDE_M/1 -> Relational Operator/1
  Bitmask_EXIDE/1 -> Relational Operator/2
  SIDL/1 -> Bitmask_EXIDE/1

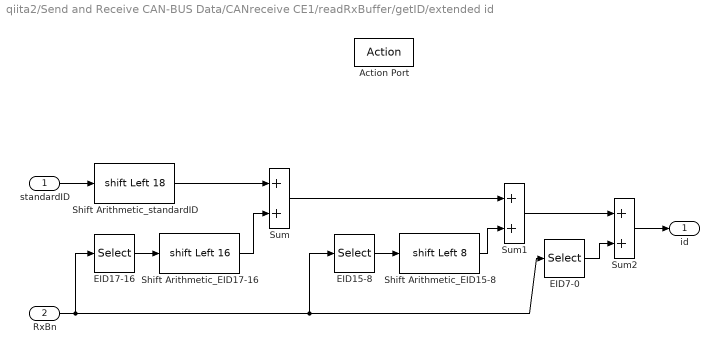
== system qiita2/Send and Receive CAN-BUS Data/CANreceive CE1/readRxBuffer/getID/extended id ==
  standardID : Inport
  RxBn : Inport  Port=2
  Action Port : ActionPort  ActionPortLabel=if(u1 == 1)
  EID15-8 : Selector  IndexMode=Zero-based  InputPortWidth=13  IndexOptions=Index vector (dialog)  Indices=2  OutputSizes=1
  EID17-16 : Selector  IndexMode=Zero-based  InputPortWidth=13  IndexOptions=Index vector (dialog)  Indices=1  OutputSizes=1
  EID7-0 : Selector  IndexMode=Zero-based  InputPortWidth=13  IndexOptions=Index vector (dialog)  Indices=3  OutputSizes=1
  Shift Arithmetic_EID15-8 : ArithShift  BitShiftNumber=8  BitShiftDirection=Left
  Shift Arithmetic_EID17-16 : ArithShift  BitShiftNumber=16  BitShiftDirection=Left
  Shift Arithmetic_standardID : ArithShift  BitShiftNumber=18  BitShiftDirection=Left
  Sum : Sum
  Sum1 : Sum
  Sum2 : Sum
  id : Outport
  wires:
  Sum2/1 -> id/1
  standardID/1 -> Shift Arithmetic_standardID/1
  Shift Arithmetic_standardID/1 -> Sum/1
  EID17-16/1 -> Shift Arithmetic_EID17-16/1
  Shift Arithmetic_EID17-16/1 -> Sum/2
  Sum/1 -> Sum1/1
  Shift Arithmetic_EID15-8/1 -> Sum1/2
  EID15-8/1 -> Shift Arithmetic_EID15-8/1
  Sum1/1 -> Sum2/1
  RxBn/1 -> EID7-0/1, EID15-8/1, EID17-16/1
  EID7-0/1 -> Sum2/2

== system qiita2/Send and Receive CAN-BUS Data/CANreceive CE1/readRxBuffer/getID/getStandardID ==
  SIDL : Inport
  SIDH : Inport  Port=2
  Bitmask_SID2-0 : simulink/Logic and Bit Operations/Bitwise Operator  logicop=AND  UseBitMask=on  BitMask=bin2dec('11100000')  BitMaskRealWorld=Stored Integer
  Data Type Conversion : DataTypeConversion  OutDataTypeStr=uint32
  Shift Arithmetic_SID10-3 : ArithShift  BitShiftNumber=3  BitShiftDirection=Left
  Shift Arithmetic_SID2-0 : ArithShift  BitShiftNumber=5  BitShiftDirection=Right
  Sum1 : Sum
  stadardID : Outport
  wires:
  Sum1/1 -> stadardID/1
  Shift Arithmetic_SID2-0/1 -> Sum1/1
  Shift Arithmetic_SID10-3/1 -> Sum1/2
  SIDL/1 -> Bitmask_SID2-0/1
  SIDH/1 -> Data Type Conversion/1
  Bitmask_SID2-0/1 -> Shift Arithmetic_SID2-0/1
  Data Type Conversion/1 -> Shift Arithmetic_SID10-3/1

== system qiita2/Send and Receive CAN-BUS Data/CANreceive CE1/readRxBuffer/getID/standard id ==
  stadardID : Inport
  Action Port : ActionPort  ActionPortLabel=else
  id : Outport
  wires:
  stadardID/1 -> id/1

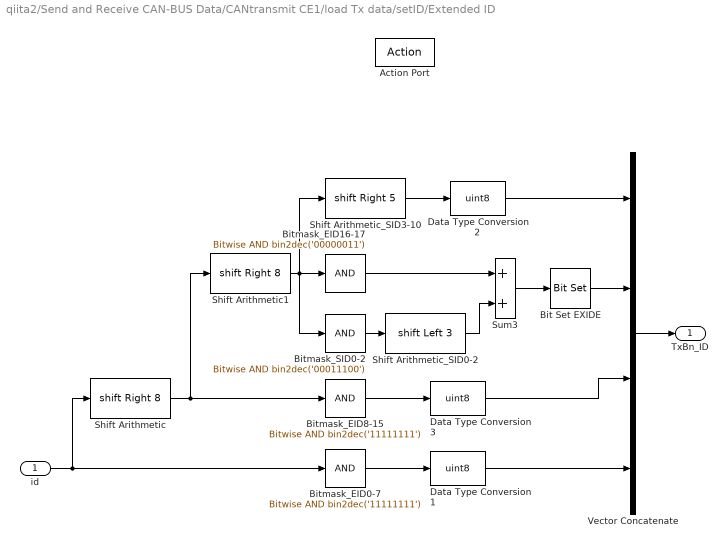
== system qiita2/Send and Receive CAN-BUS Data/CANtransmit CE1/load Tx data/setID/Extended ID ==
  id : Inport
  Action Port : ActionPort  ActionPortLabel=if(u1 > 0)
  Bit Set EXIDE : simulink/Logic and Bit Operations/Bit Set  iBit=3
      settings: SourceProductName=Simulink  SourceProductBaseCode=SL
  Bitmask_EID0-7 : simulink/Logic and Bit Operations/Bitwise Operator  logicop=AND  UseBitMask=on  BitMask=bin2dec('11111111')  BitMaskRealWorld=Stored Integer
  Bitmask_EID16-17 : simulink/Logic and Bit Operations/Bitwise Operator  logicop=AND  UseBitMask=on  BitMask=bin2dec('00000011')  BitMaskRealWorld=Stored Integer
  Bitmask_EID8-15 : simulink/Logic and Bit Operations/Bitwise Operator  logicop=AND  UseBitMask=on  BitMask=bin2dec('11111111')  BitMaskRealWorld=Stored Integer
  Bitmask_SID0-2 : simulink/Logic and Bit Operations/Bitwise Operator  logicop=AND  UseBitMask=on  BitMask=bin2dec('00011100')  BitMaskRealWorld=Stored Integer
  Data Type Conversion1 : DataTypeConversion  OutDataTypeStr=uint8  RndMeth=Simplest
  Data Type Conversion2 : DataTypeConversion  OutDataTypeStr=uint8  RndMeth=Simplest
  Data Type Conversion3 : DataTypeConversion  OutDataTypeStr=uint8  RndMeth=Simplest
  Shift Arithmetic : ArithShift  BitShiftNumber=8  BitShiftDirection=Right
  Shift Arithmetic1 : ArithShift  BitShiftNumber=8  BitShiftDirection=Right
  Shift Arithmetic_SID0-2 : ArithShift  BitShiftNumber=3  BitShiftDirection=Left
  Shift Arithmetic_SID3-10 : ArithShift  BitShiftNumber=5  BitShiftDirection=Right
  Sum3 : Sum  OutDataTypeStr=uint8
  Vector Concatenate : Concatenate  NumInputs=4
  TxBn_ID : Outport
  wires:
  Vector Concatenate/1 -> TxBn_ID/1
  id/1 -> Shift Arithmetic/1, Bitmask_EID0-7/1
  Bitmask_EID0-7/1 -> Data Type Conversion1/1
  Data Type Conversion1/1 -> Vector Concatenate/4
  Shift Arithmetic/1 -> Shift Arithmetic1/1, Bitmask_EID8-15/1
  Bitmask_EID8-15/1 -> Data Type Conversion3/1
  Data Type Conversion3/1 -> Vector Concatenate/3
  Shift Arithmetic1/1 -> Shift Arithmetic_SID3-10/1, Bitmask_SID0-2/1, Bitmask_EID16-17/1
  Sum3/1 -> Bit Set EXIDE/1
  Bitmask_EID16-17/1 -> Sum3/1
  Bitmask_SID0-2/1 -> Shift Arithmetic_SID0-2/1
  Shift Arithmetic_SID0-2/1 -> Sum3/2
  Bit Set EXIDE/1 -> Vector Concatenate/2
  Shift Arithmetic_SID3-10/1 -> Data Type Conversion2/1
  Data Type Conversion2/1 -> Vector Concatenate/1

== system qiita2/Send and Receive CAN-BUS Data/CANtransmit CE1/load Tx data/setID/Standard ID ==
  id : Inport
  Action Port : ActionPort  ActionPortLabel=else
  Vector Concatenate : Concatenate  NumInputs=4
  convert_ID : Subsystem  TreatAsAtomicUnit=on
  no data : Constant  Value=0  OutDataTypeStr=uint8
  TxBn_ID : Outport
  wires:
  Vector Concatenate/1 -> TxBn_ID/1
  no data/1 -> Vector Concatenate/3, Vector Concatenate/4
  convert_ID/2(SIDL) -> Vector Concatenate/2
  id/1 -> convert_ID/1(id)
  convert_ID/1(SIDH) -> Vector Concatenate/1

== system qiita2/Send and Receive CAN-BUS Data/CANtransmit CE1/load Tx data/setID/Standard ID/convert_ID ==
  id : Inport
  Bitmask_SID0-10 : simulink/Logic and Bit Operations/Bitwise Operator  logicop=AND  UseBitMask=on  BitMask=bin2dec('0000011111111111')  BitMaskRealWorld=Stored Integer
  Bitmask_SID0-2 : simulink/Logic and Bit Operations/Bitwise Operator  logicop=AND  UseBitMask=on  BitMask=bin2dec('0000000011100000')  BitMaskRealWorld=Stored Integer
  Data Type Conversion1 : DataTypeConversion  OutDataTypeStr=uint8  RndMeth=Simplest
  Data Type Conversion2 : DataTypeConversion  OutDataTypeStr=uint8  RndMeth=Simplest
  Shift Arithmetic1 : ArithShift  BitShiftNumber=3  BitShiftDirection=Right
  Shift Arithmetic2 : ArithShift  BitShiftNumber=5  BitShiftDirection=Left
  SIDH : Outport
  SIDL : Outport  Port=2
  wires:
  Shift Arithmetic1/1 -> Data Type Conversion1/1
  Data Type Conversion1/1 -> SIDH/1
  Bitmask_SID0-10/1 -> Shift Arithmetic2/1, Shift Arithmetic1/1
  Data Type Conversion2/1 -> SIDL/1
  Shift Arithmetic2/1 -> Bitmask_SID0-2/1
  id/1 -> Bitmask_SID0-10/1
  Bitmask_SID0-2/1 -> Data Type Conversion2/1
